simulink model "mcb_open_loop_control_f28035_DRV8312"  (R2021b)
settings: Solver=FixedStepDiscrete  StartTime=0.0  StopTime=Inf  RelTol=1e-3  EnableMultiTasking=on
InitFcn:
  | mcb_c2000_open_loop_control_data;
  | target = mcb_SetProcessorDetails('F28035',PWM_frequency);
model workspace (MAT data in the model file):
  encoderResolution = 2000
  hallOffset = '0.5'
  indexOffset = 850
  polePairs = '4'
values from neighbouring files (symbols this model uses):
  PWM_frequency = 20e3    (= 20000)    [c28027pmsmfoc_data.m]    (also in c28035pmsmfoc_data.m; c28035pmsmfoc_data_cla.m = 12000; c28069pmsmfoc_data.m; mcb_c2000_open_loop_control_data.m = eval(get_param([bdroot '/Open Loop Control/Parameters/PWM Fr)
  Ts = 5e-8    (= 5e-08)    [DCDC_Buck_Param.m]    (also in mcb_c2000_open_loop_control_data.m = T_pwm; mcb_c2000_pmsm_offset_data.m = T_pwm; mcb_pmsm_foc_dual_f28379d_data.m = 5e-05; mcb_pmsm_foc_dual_f28379d_datascript.m = 5e-05)
undefined symbols (not defined in the file or in its folder): DiscIntNeverNeededParam, Down, GPTRIP1SEL, GPTRIP2SEL, motor, TZ1, TZ2, Up
libraries: c2802xlib x4, simulink x3, mcbcontrolslib x3, c2803xlib x2, c280xlib x2, c2000lib x1, demo_controls x1
settings Model: ExtModeTrigDuration=8  Creator=The MathWorks, Inc.  LastModifiedBy=The MathWorks, Inc.
settings SolverCC: AlgebraicLoopSolver=TrustRegion  AutoInsertRateTranBlk=on
settings DataIOCC: LimitDataPoints=on  SaveFormat=Array  SaveOutput=off  SaveTime=off  ReturnWorkspaceOutputs=off
settings OptimizationCC: DefaultParameterBehavior=Inlined  DefaultUnderspecifiedDataType=single  OptimizeBlockIOStorage=off  BufferReuse=off  GlobalBufferReuse=off  ExpressionFolding=off  ExpressionDepthLimit=2147483647  LocalBlockOutputs=off  InitFltsAndDblsToZero=on  NoFixptDivByZeroProtection=on  EfficientFloat2IntCast=on  EfficientMapNaN2IntZero=off  LifeSpan=Inf  MaxStackSize=768  OptimizeDataStoreBuffers=off  BusAssignmentInplaceUpdate=off  DenormalBehavior=FlushToZero  EfficientTunableParamExpr=on
settings DebuggingCC: ReadBeforeWriteMsg=DisableAll  WriteAfterWriteMsg=DisableAll  WriteAfterReadMsg=DisableAll  CheckSSInitialOutputMsg=off  SignalResolutionControl=TryResolveAllWithWarning  SolverPrmCheckMsg=warning  InheritedTsInSrcMsg=none  MultiTaskDSMMsg=none  MultiTaskCondExecSysMsg=none  TasksWithSamePriorityMsg=none  SigSpecEnsureSampleTimeMsg=none  IntegerOverflowMsg=none  ParameterPrecisionLossMsg=none  FcnCallInpInsideContextMsg=warning  AllowSymbolicDim=off  StateNameClashWarn=warning  SFUnexpectedBacktrackingDiag=warning  SFNoUnconditionalDefaultTransitionDiag=warning  SFExecutionAtInitializationDiag=none  SFMachineParentedDataDiag=warning  IntegerSaturationMsg=none  ArithmeticOperatorsInVariantConditions=warning
settings HardwareCC: ProdBitPerChar=16  ProdBitPerInt=16  ProdBitPerPointer=32  ProdBitPerSizeT=32  ProdBitPerPtrDiffT=32  ProdLargestAtomicInteger=Integer  ProdLargestAtomicFloat=None  ProdWordSize=16  ProdLongLongMode=on  ProdHWDeviceType=Texas Instruments->C2000  TargetBitPerChar=16  TargetBitPerInt=16  TargetBitPerPointer=16  TargetLargestAtomicInteger=Integer  TargetIntDivRoundTo=Zero  TargetEndianess=LittleEndian  TargetWordSize=16  TargetHWDeviceType=TI C2000
settings ModelReferenceCC: PropagateSignalLabelsOutOfModel=off
settings SFSimCC: SimUseLocalCustomCode=off  MATLABDynamicMemAlloc=off  CustomCodeUndefinedFunction=UseInterfaceOnly
settings RTWCC: Description=Embedded Coder  SystemTargetFile=ert.tlc  HardwareBoard=TI Piccolo F2803x  TemplateMakefile=ert_default_tmf  GenerateReport=on  RTWUseLocalCustomCode=off  Toolchain=Texas Instruments Code Composer Studio (C2000)  IncludeHyperlinkInReport=on  GenerateTraceInfo=on  GenerateTraceReport=on  GenerateTraceReportSl=on  GenerateTraceReportSf=on  GenerateTraceReportEml=on
settings CodeAppCC: IgnoreCustomStorageClasses=off  CustomSymbolStrType=$N$R$M  StateflowObjectComments=on  InternalIdentifier=Classic
settings ERTTargetCC: CodeReplacementLibrary=TI C28x  MultiwordLength=2048  ExtModeTransport=3  ExtModeStaticAllocSize=1000  ConvertIfToSwitch=off  SuppressUnreachableDefaultCases=off  MemSecPackage=tic2000demospkg
settings ConfigComp: CovMetricSettings=dw  CovSaveCumulativeToWorkspaceVar=on  CovSaveSingleToWorkspaceVar=on  CovExternalEMLEnable=off  CovSFcnEnable=off

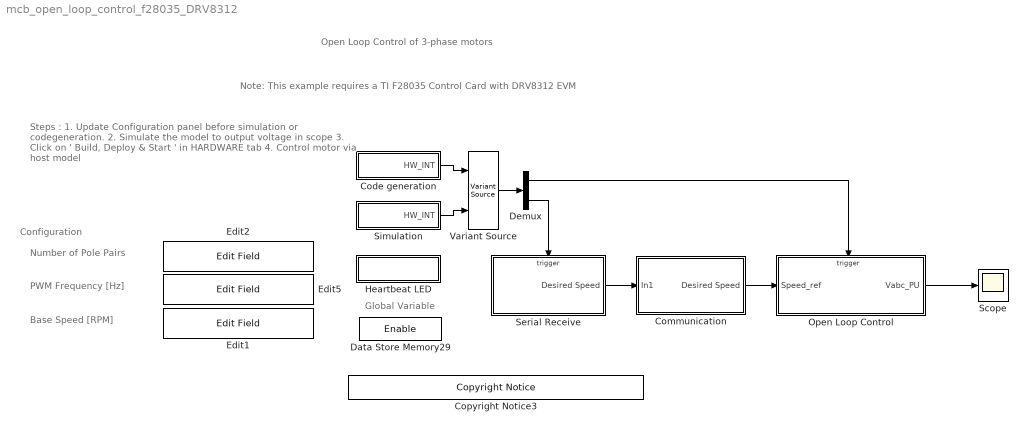
== system mcb_open_loop_control_f28035_DRV8312 ==
  note: Global Variable
  note: Open Loop Control of 3-phase motors
  note: Note: This example requires a TI F28035 Control Card with DRV8312 EVM
  note: Base Speed [RPM]
  note: Number of Pole Pairs
  note: Configuration
  note: PWM Frequency [Hz]
  note: Steps :
      | 1. Update Configuration panel before simulation or
      | codegeneration.
      | 2. Simulate the model to output voltage in scope
      | 3. Click on ' Build, Deploy & Start ' in HARDWARE tab
      | 4. Control motor via host model
  Code generation : Subsystem
  Communication : Subsystem
  Copyright Notice3 : demo_controls/Copyright Notice  year=2021  prod=tic2000
      settings: SourceProductBaseCode=ME
  Data Store Memory29 : DataStoreMemory  DataStoreName=Enable  ShowAdditionalParam=off  OutDataTypeStr=boolean
  Demux : Demux  Outputs=2
  Edit1 : EditField  LabelPosition=Hide  ShowInitialText=on  Alignment=Center
  Edit2 : EditField  LabelPosition=Hide  ShowInitialText=on  Alignment=Center
  Edit5 : EditField  LabelPosition=Hide  ShowInitialText=on  Alignment=Center
  Heartbeat LED : Subsystem  TreatAsAtomicUnit=on
  Open Loop Control : Subsystem
      settings: RTWSystemCode=Nonreusable function
  Scope : Scope
  Serial Receive : Subsystem  SystemSampleTime=1e-3
      settings: RTWSystemCode=Nonreusable function
  Simulation : Subsystem
  Variant Source : VariantSource  VariantControlMode=sim codegen switching  OutputFunctionCall=on
  wires:
  Demux/2 -> Serial Receive/Trigger
  Demux/1 -> Open Loop Control/Trigger
  Open Loop Control/1(Vabc_PU) -> Scope/1
  Code generation/1(HW_INT) -> Variant Source/1
  Simulation/1(HW_INT) -> Variant Source/2
  Variant Source/1 -> Demux/1
  Communication/1(Desired Speed) -> Open Loop Control/1(Speed_ref)
  Serial Receive/1(Desired Speed) -> Communication/1(In1)

== system mcb_open_loop_control_f28035_DRV8312/Code generation ==
  C28x Hardware Interrupt : c2000lib/Scheduling/C28x Hardware Interrupt  irqnumbers=[1 9]  pienumbers=[1 1]  irqpriorities=[30 50]  irqpreempts=[1 0]  showinput=off  dspchiptype=C280X
      settings: SourceProductBaseCode=TIC2000
  HW_INT : Outport
  wires:
  C28x Hardware Interrupt/1 -> HW_INT/1

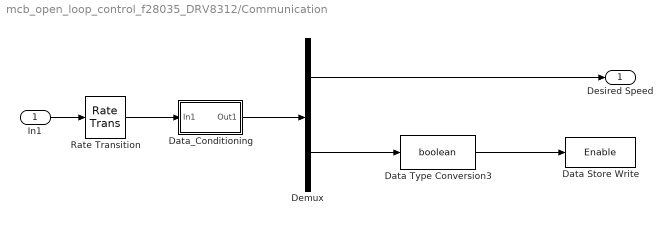
== system mcb_open_loop_control_f28035_DRV8312/Communication ==
  In1 : Inport
  Data Store Write : DataStoreWrite  DataStoreName=Enable  IndexOptions=Index vector (dialog)  Indices=1  OutputSizes=1
  Data Type Conversion3 : DataTypeConversion  OutDataTypeStr=boolean  RndMeth=Simplest
  Data_Conditioning : Subsystem
  Demux : Demux  Outputs=2
  Rate Transition : RateTransition  Deterministic=off  InitialCondition=[1228 0]  OutPortSampleTime=Ts
  Desired Speed : Outport  VectorParamsAs1DForOutWhenUnconnected=off
  wires:
  Rate Transition/1 -> Data_Conditioning/1(In1)
  In1/1 -> Rate Transition/1
  Data_Conditioning/1(Out1) -> Demux/1
  Demux/2 -> Data Type Conversion3/1
  Demux/1 -> Desired Speed/1
  Data Type Conversion3/1 -> Data Store Write/1

== system mcb_open_loop_control_f28035_DRV8312/Heartbeat LED ==
  Code generation : Subsystem
  LED 1 Hz : Constant  OutDataTypeStr=uint16  SampleTime=0.5
  Simulation : Subsystem
  Variant Sink : VariantSink  VariantControlMode=sim codegen switching
  wires:
  Variant Sink/1 -> Code generation/1(In1)
  Variant Sink/2 -> Simulation/1(In1)
  LED 1 Hz/1 -> Variant Sink/1

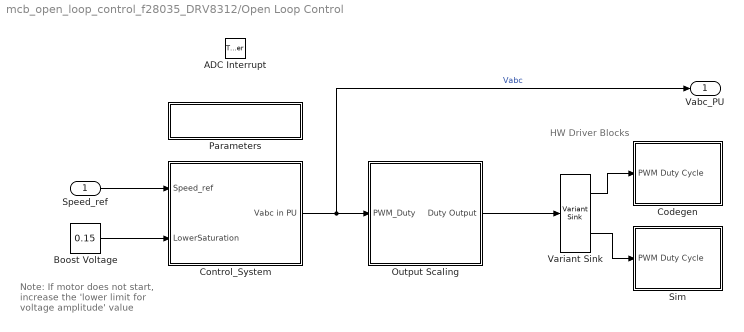
== system mcb_open_loop_control_f28035_DRV8312/Open Loop Control ==
  note: Note: If motor does not start, increase the 'lower limit for voltage amplitude' value
  note: HW Driver Blocks
  Speed_ref : Inport
  ADC Interrupt : TriggerPort  TriggerType=function-call  VariantControl=Variant
  Boost Voltage : Constant  Value=0.15  OutDataTypeStr=dataType
  Codegen : Subsystem
  Control_System : Subsystem
  Output Scaling : Subsystem
  Parameters : Subsystem
  Sim : Subsystem
  Variant Sink : VariantSink  VariantControlMode=sim codegen switching
  Vabc_PU : Outport  VectorParamsAs1DForOutWhenUnconnected=off
  wires:
  Speed_ref/1 -> Control_System/1(Speed_ref)
  Control_System/1(Vabc in PU) -> Vabc_PU/1, Output Scaling/1(PWM_Duty)  "Vabc"
  Output Scaling/1(Duty Output) -> Variant Sink/1
  Variant Sink/1 -> Codegen/1(PWM Duty Cycle)
  Variant Sink/2 -> Sim/1(PWM Duty Cycle)
  Boost Voltage/1 -> Control_System/2(LowerSaturation)

== system mcb_open_loop_control_f28035_DRV8312/Serial Receive ==
  SCI_Rx_INT : TriggerPort  TriggerType=function-call  VariantControl=Variant
  Codegen : Subsystem
  Sim : Subsystem
  Variant Source : VariantSource  VariantControlMode=sim codegen switching
  Desired Speed : Outport  VectorParamsAs1DForOutWhenUnconnected=off
  wires:
  Variant Source/1 -> Desired Speed/1
  Codegen/1(Output) -> Variant Source/1
  Sim/1(Out1) -> Variant Source/2

== system mcb_open_loop_control_f28035_DRV8312/Simulation ==
  ADCINT1 : simulink/Ports & Subsystems/Function-Call Generator  sample_time=Ts  numberOfIterations=1  DisallowWideOutput=off
  Mux : Mux  Inputs=2
  SCI_Rx_INT : simulink/Ports & Subsystems/Function-Call Generator  sample_time=0.1  numberOfIterations=1  DisallowWideOutput=off
  HW_INT : Outport
  wires:
  SCI_Rx_INT/1 -> Mux/2
  ADCINT1/1 -> Mux/1
  Mux/1 -> HW_INT/1

== system mcb_open_loop_control_f28035_DRV8312/Communication/Data_Conditioning ==
  In1 : Inport
  Data Type Conversion2 : DataTypeConversion  OutDataTypeStr=int16  ConvertRealWorld=Stored Integer (SI)  RndMeth=Simplest
  Out1 : Outport  VectorParamsAs1DForOutWhenUnconnected=off
  wires:
  Data Type Conversion2/1 -> Out1/1
  In1/1 -> Data Type Conversion2/1

== system mcb_open_loop_control_f28035_DRV8312/Heartbeat LED/Code generation ==
  In1 : Inport
  Digital Output1 : c2803xlib/Digital Output  GPIO_Number=GPIO24~GPIO31  GPIO_Bit0=off  GPIO_BIT0_Toggle=off  GPIO_Bit1=off  GPIO_BIT1_Toggle=off  GPIO_Bit2=off  GPIO_BIT2_Toggle=off  GPIO_Bit3=off  GPIO_BIT3_Toggle=off  GPIO_Bit4=off  GPIO_BIT4_Toggle=off  GPIO_Bit5=off  GPIO_BIT5_Toggle=off  GPIO_Bit6=off  GPIO_BIT6_Toggle=off  GPIO_Bit7=on  GPIO_BIT7_Toggle=on
      settings: SourceProductBaseCode=TIC2000
  wires:
  In1/1 -> Digital Output1/1

== system mcb_open_loop_control_f28035_DRV8312/Heartbeat LED/Simulation ==
  In1 : Inport
  Simulation_Terminator : Terminator
  wires:
  In1/1 -> Simulation_Terminator/1

== system mcb_open_loop_control_f28035_DRV8312/Open Loop Control/Codegen ==
  PWM Duty Cycle : Inport
  Data Serial Output : Subsystem
  Demux : Demux  Outputs=2
  Hardware Initialization : Subsystem
  PWM Output : Subsystem
  Sensors : Subsystem
  wires:
  Demux/2 -> Data Serial Output/2(Data2_Log)
  Sensors/1(Iab_measured_ADC) -> Demux/1
  Demux/1 -> Data Serial Output/1(Data1_Log)
  PWM Duty Cycle/1 -> PWM Output/1(PWM Duty Cycle)

== system mcb_open_loop_control_f28035_DRV8312/Open Loop Control/Control_System ==
  Speed_ref : Inport
  LowerSaturation : Inport  Port=2
  SpeedRefToFreq : Subsystem
  VabcCalc : Subsystem
  Vabc in PU : Outport  VectorParamsAs1DForOutWhenUnconnected=off
  wires:
  Speed_ref/1 -> SpeedRefToFreq/1(Speed_Ref)
  SpeedRefToFreq/1(Frequency) -> VabcCalc/1(Frequency)
  VabcCalc/1(Vabc) -> Vabc in PU/1
  LowerSaturation/1 -> VabcCalc/2(LowerSaturation)

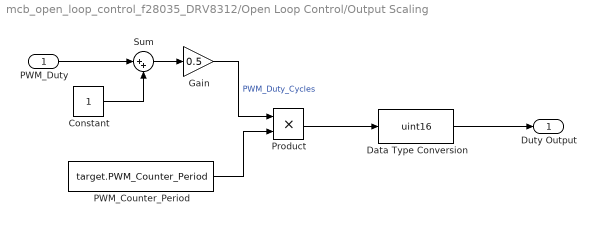
== system mcb_open_loop_control_f28035_DRV8312/Open Loop Control/Output Scaling ==
  PWM_Duty : Inport
  Constant : Constant  OutDataTypeStr=dataType
  Data Type Conversion : DataTypeConversion  OutDataTypeStr=uint16  SaturateOnIntegerOverflow=on
  Gain : Gain  Gain=0.5  RndMeth=Simplest  OutDataTypeStr=Inherit: Same as input
  PWM_Counter_Period : Constant  Value=target.PWM_Counter_Period  OutDataTypeStr=dataType  SampleTime=-1
  Product : Product  RndMeth=Simplest  OutDataTypeStr=Inherit: Same as first input
  Sum : Sum  Inputs=|++
  Duty Output : Outport
  wires:
  Data Type Conversion/1 -> Duty Output/1
  PWM_Counter_Period/1 -> Product/2
  PWM_Duty/1 -> Sum/1
  Product/1 -> Data Type Conversion/1
  Constant/1 -> Sum/2
  Sum/1 -> Gain/1
  Gain/1 -> Product/1  "PWM_Duty_Cycles"

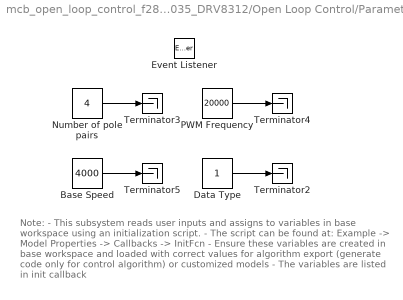
== system mcb_open_loop_control_f28035_DRV8312/Open Loop Control/Parameters ==
  note: Note:
      | - This subsystem reads user inputs and assigns to variables
      | in base workspace using an initialization script.
      | - The script can be found at: Example -> Model Properties ->
      | Callbacks -> InitFcn
      | - Ensure these variables are created in base workspace and
      | loaded with correct values for algorithm export (generate
      | code only for control algorithm) or customized models
      | - The variables are listed in init callback
  Base Speed : Constant  Value=4000
  Data Type : Constant
  Event Listener : EventListener  DisableCoverage=on  EventName=reset
  Number of pole pairs : Constant  Value=4
  PWM Frequency : Constant  Value=20000
  Terminator{2..5} (4 alike) : Terminator
  wires:
  Data Type/1 -> Terminator2/1
  Number of pole pairs/1 -> Terminator3/1
  PWM Frequency/1 -> Terminator4/1
  Base Speed/1 -> Terminator5/1

== system mcb_open_loop_control_f28035_DRV8312/Open Loop Control/Sim ==
  PWM Duty Cycle : Inport
  Terminator : Terminator
  wires:
  PWM Duty Cycle/1 -> Terminator/1

== system mcb_open_loop_control_f28035_DRV8312/Serial Receive/Codegen ==
  SCI Receive : c280xlib/SCI Receive  sciModule=A  dataHead=''  dataTail=''  dataType=uint16  dataDim=2  initValue=0  errOption=Output the last received value  errValue=0  sampleTime=-1  outputStatus=off  postInterrupt=on  numFifo=4
      settings: SourceProductBaseCode=TIC2000
  Output : Outport
  wires:
  SCI Receive/1 -> Output/1

== system mcb_open_loop_control_f28035_DRV8312/Serial Receive/Sim ==
  Constant : Constant  OutDataTypeStr=dataType
  Data Type Conversion : DataTypeConversion  OutDataTypeStr=int16
  Data Type Conversion3 : DataTypeConversion  OutDataTypeStr=uint16  ConvertRealWorld=Stored Integer (SI)  RndMeth=Simplest
  Mux : Mux  Inputs=2
  Speed_ref_rpm (sim) : Constant  Value=1200  OutDataTypeStr=dataType  SampleTime=-1
  Out1 : Outport
  wires:
  Data Type Conversion3/1 -> Out1/1
  Mux/1 -> Data Type Conversion/1
  Constant/1 -> Mux/2
  Speed_ref_rpm (sim)/1 -> Mux/1
  Data Type Conversion/1 -> Data Type Conversion3/1

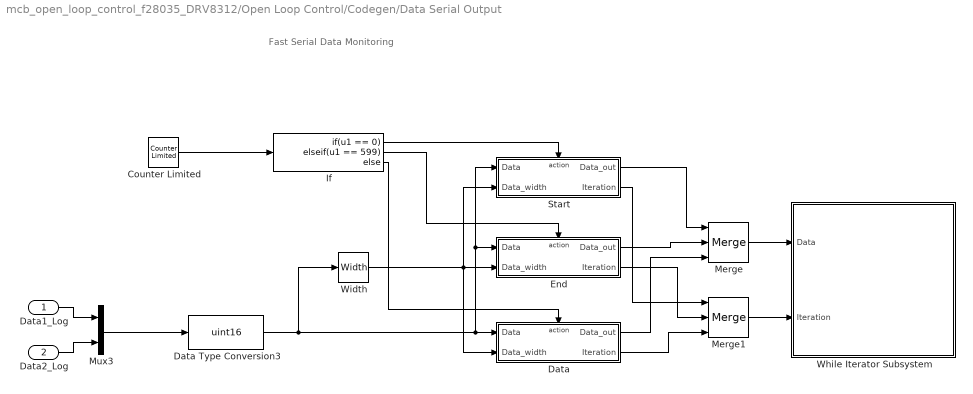
== system mcb_open_loop_control_f28035_DRV8312/Open Loop Control/Codegen/Data Serial Output ==
  note: Fast Serial Data Monitoring
  Data1_Log : Inport
  Data2_Log : Inport  Port=2
  Counter Limited : simulink/Sources/Counter Limited  uplimit=599  tsamp=-1
  Data : Subsystem  TreatAsAtomicUnit=on
  Data Type Conversion3 : DataTypeConversion  OutDataTypeStr=uint16  ConvertRealWorld=Stored Integer (SI)
  End : Subsystem  TreatAsAtomicUnit=on
  If : If  IfExpression=u1 == 0  ElseIfExpressions=u1 == 599
  Merge : Merge  Inputs=3
  Merge1 : Merge  Inputs=3
  Mux3 : Mux  Inputs=2
  Start : Subsystem  TreatAsAtomicUnit=on
  While Iterator Subsystem : Subsystem  TreatAsAtomicUnit=on
  Width : Width  OutDataTypeMode=All ports same datatype  DataType=uint16
  wires:
  Merge/1 -> While Iterator Subsystem/1(Data)
  If/2 -> End/Action
  If/3 -> Data/Action
  Counter Limited/1 -> If/1
  End/1(Data_out) -> Merge/2
  Width/1 -> Data/2(Data_width), Start/2(Data_width), End/2(Data_width)
  Start/1(Data_out) -> Merge/1
  Start/2(Iteration) -> Merge1/1
  Merge1/1 -> While Iterator Subsystem/2(Iteration)
  Data/1(Data_out) -> Merge/3
  If/1 -> Start/Action
  End/2(Iteration) -> Merge1/2
  Data/2(Iteration) -> Merge1/3
  Data Type Conversion3/1 -> Width/1, Start/1(Data), End/1(Data), Data/1(Data)
  Data2_Log/1 -> Mux3/2
  Data1_Log/1 -> Mux3/1
  Mux3/1 -> Data Type Conversion3/1

== system mcb_open_loop_control_f28035_DRV8312/Open Loop Control/Codegen/Hardware Initialization ==
  Data Store Read1 : DataStoreRead  DataStoreName=Enable  IndexOptions=Index vector (dialog)  Indices=1  OutputSizes=1
  Digital Output : c2803xlib/Digital Output  GPIO_Number=GPIO0~GPIO7  GPIO_Bit0=off  GPIO_BIT0_Toggle=off  GPIO_Bit1=on  GPIO_BIT1_Toggle=off  GPIO_Bit2=off  GPIO_BIT2_Toggle=off  GPIO_Bit3=on  GPIO_BIT3_Toggle=off  GPIO_Bit4=off  GPIO_BIT4_Toggle=off  GPIO_Bit5=on  GPIO_BIT5_Toggle=off  GPIO_Bit6=off  GPIO_BIT6_Toggle=off  GPIO_Bit7=off  GPIO_BIT7_Toggle=off
      settings: SourceProductBaseCode=TIC2000
  Mux : Mux  Inputs=3
  wires:
  Mux/1 -> Digital Output/1
  Data Store Read1/1 -> Mux/3, Mux/2, Mux/1

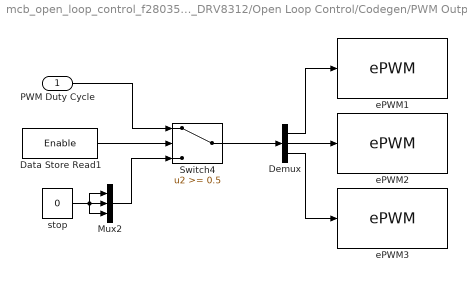
== system mcb_open_loop_control_f28035_DRV8312/Open Loop Control/Codegen/PWM Output ==
  PWM Duty Cycle : Inport
  Data Store Read1 : DataStoreRead  DataStoreName=Enable  IndexOptions=Index vector (dialog)  Indices=1  OutputSizes=1
  Demux : Demux  Outputs=3
  Mux2 : Mux  Inputs=3
  Switch4 : Switch  Threshold=0.5  RndMeth=Simplest
  ePWM1 : c2802xlib/ePWM  PwmType=C2000  useModule=ePWM1  ePWMxLINKTBPRD=Not Linked  periodUnits=Clock cycles  timerSource=Specify via dialog  timerPeriod_clk=target.PWM_Counter_Period+1  timerPeriod_sec=64000  tbshadow=Counter equals to zero  countingMode=Up-Down  phaseActiveEnable=Disable  phaseDirection=Count down after sync  phaseActive=0  synchronizationEnable=off  dcaevt1Sync=off  dcbevt1Sync=off  synchronizationOption=Counter equals to zero (CTR=Zero)  perSynchronizationOption=Counter equals to period (CTR=PRD)  clockPrescale=1  HSclockPrescale=1  enswap=off  ePWMxAStatus=on  ePWMxAactionLogic1=Do nothing  ePWMxAactionLogic2=Do nothing  ePWMxAactionLogic3=Clear  ePWMxAactionLogic4=Set  ePWMxAactionLogic5=Do nothing  ePWMxAactionLogic6=Do nothing  ePWMxACSFenable=off  ePWMxACSFvalue=Forcing disable  ePWMxASFreload=Zero  ePWMxBStatus=off  ePWMxBactionLogic1=Do nothing  ePWMxBactionLogic2=Set  ePWMxBactionLogic3=Do nothing  ePWMxBactionLogic4=Do nothing  ePWMxBactionLogic5=Clear  ePWMxBactionLogic6=Do nothing  ePWMxBCSFenable=off  ePWMxBCSFvalue=Forcing disable  ePWMxBSFreload=Zero  ePWNxBOutWay=off  ePWMxLINKCMPA=Not Linked  CMPAUnits=Clock cycles  CMPASource=Input port  CMPAValue_per=32000  CMPAValue_clk=target.PWM_Counter_Period/2+1  enCMPAshadow=Counter equals to zero (CTR=Zero)  ePWMxLINKCMPB=Not Linked  CMPBUnits=Clock cycles  CMPBSource=Specify via dialog  CMPBValue_per=50  CMPBValue_clk=target.PWM_Counter_Period/2+1  enCMPBshadow=Counter equals to zero (CTR=Zero)  ePWMxLINKCMPC=Not Linked  CMPCUnits=Clock cycles  CMPCSource=Specify via dialog  CMPCValue_per=50  CMPCValue_clk=32000  enCMPCshadow=Counter equals to zero (CTR=Zero)  ePWMxLINKCMPD=Not Linked  CMPDUnits=Clock cycles  CMPDSource=Specify via dialog  CMPDValue_per=50  CMPDValue_clk=32000  enCMPDshadow=Counter equals to zero (CTR=Zero)  enableDBePWMxA=off  enableDBePWMxB=off  enhalfcycle=off  DBpolarity=Active high (AH)  DBedgeDelay=Positive  DBSource_ePWMxA=ePWMxA  DBSource_ePWMxB=ePWMxA  DBPeriodUnits=Clock cycles  DBperiodSource=Specify via dialog  REDperiod=0  FEDperiod=0  REDperiod_sec=0  FEDperiod_sec=0  LoadModeDBRED=Immediate without using shadow  LoadModeDBFED=Immediate without using shadow  adcstartModuleA=on  adcrequestEventA=First event  adcstartEventA=Counter equals to period (CTR=PRD)  adcstartEventA_type2=Digital Compare Module A Event 1 start of conversion (DCAEVT1.soc)  adcstartModuleB=off  adcrequestEventB=First event  adcstartEventB=Counter equals to zero (CTR=Zero)  adcstartEventB_type2=Counter equals to zero (CTR=Zero)  intEn=off  intPrd=First event  intSel=Counter equals to zero (CTR=Zero)  intSel_type2=Counter equals to zero (CTR=Zero)  hrpe=off  enHRPWM=off  HRPWM_LoadMode=Counter equals to period (CTR=PRD)  HRPWM_CTLMode=Duty or Period control mode  HRPWM_EDGMode=Both edge  hrpeb=off  enHRPWMB=off  HRPWM_LoadModeB=Counter equals to zero (CTR=ZERO)  HRPWM_CTLModeB=Duty or Period control mode  HRPWM_EDGModeB=Both edge  enHRDBRED=off  enHRDBFED=off  enSFO=on  enautoconv=on  chopperEnable=off  chopperFrequency=1  chopperFirstwidth=1  chopperDuty=12.5%  tripZonesource=Specify via dialog  tzselOSHT1=off  tzselOSHT2=off  tzselOSHT3=off  tzselOSHDCAEV1=off  tzselOSHDCBEV1=off  tzselCBC1=off  tzselCBC2=off  tzselCBC3=off  tzselCBCDCAEV2=off  tzselCBCDCBEV2=off  tzselOSHT4=off  tzselOSHT5=off  tzselOSHT6=off  tzselCBC4=off  tzselCBC5=off  tzselCBC6=off  enTzOstIntr=off  enTzCbcIntr=off  enTzDCAEVT1Intr=off  enTzDCAEVT2Intr=off  enTzDCBEVT1Intr=off  enTzDCBEVT2Intr=off  ePWMxAforced=No action  ePWMxBforced=No action  DCAEVT1forced=No action  DCBEVT1forced=No action  DCAEVT2forced=No action  DCBEVT2forced=No action  dcah=Trip Zone 1 input (TZ1)  dcal=Trip Zone 2 input (TZ2)  dcbh=Trip Zone 1 input (TZ1)  dcbl=Trip Zone 2 input (TZ2)  dcah_type2=GPTRIP1SEL/(TZ1)  dcal_type2=GPTRIP2SEL/(TZ2)  dcbh_type2=GPTRIP1SEL/(TZ1)  dcbl_type2=GPTRIP2SEL/(TZ2)  gendcaevt1=Event disabled  gendcaevt2=Event disabled  gendcbevt1=Event disabled  gendcbevt2=Event disabled  dcaevt1src=DCAEVT1 with sync  dcaevt2src=DCAEVT2 with sync  dcbevt1src=DCBEVT1 with sync  dcbevt2src=DCBEVT2 with sync  pulsesel=Counter equals to zero (CTR=Zero)  blankinv=off  blankoffset=0  blankwidth=0  evsrcsel=Filtered version of DCAEVT1 (DCAEVT1FILT)  encape=off
  ePWM2 : c2802xlib/ePWM  PwmType=C2000  useModule=ePWM2  ePWMxLINKTBPRD=Not Linked  periodUnits=Clock cycles  timerSource=Specify via dialog  timerPeriod_clk=target.PWM_Counter_Period+1  timerPeriod_sec=64000  tbshadow=Counter equals to zero  countingMode=Up-Down  phaseActiveEnable=Set counter to phase value specified via dialog  phaseDirection=Count up after sync  phaseActive=0  synchronizationEnable=off  dcaevt1Sync=off  dcbevt1Sync=off  synchronizationOption=Pass through (EPWMxSYNCI or SWFSYNC)  perSynchronizationOption=Counter equals to period (CTR=PRD)  clockPrescale=1  HSclockPrescale=1  enswap=off  ePWMxAStatus=on  ePWMxAactionLogic1=Do nothing  ePWMxAactionLogic2=Do nothing  ePWMxAactionLogic3=Clear  ePWMxAactionLogic4=Set  ePWMxAactionLogic5=Do nothing  ePWMxAactionLogic6=Do nothing  ePWMxACSFenable=off  ePWMxACSFvalue=Forcing disable  ePWMxASFreload=Zero  ePWMxBStatus=off  ePWMxBactionLogic1=Do nothing  ePWMxBactionLogic2=Set  ePWMxBactionLogic3=Do nothing  ePWMxBactionLogic4=Do nothing  ePWMxBactionLogic5=Clear  ePWMxBactionLogic6=Do nothing  ePWMxBCSFenable=off  ePWMxBCSFvalue=Forcing disable  ePWMxBSFreload=Zero  ePWNxBOutWay=off  ePWMxLINKCMPA=Not Linked  CMPAUnits=Clock cycles  CMPASource=Input port  CMPAValue_per=32000  CMPAValue_clk=target.PWM_Counter_Period/2+1  enCMPAshadow=Counter equals to zero (CTR=Zero)  ePWMxLINKCMPB=Not Linked  CMPBUnits=Clock cycles  CMPBSource=Specify via dialog  CMPBValue_per=50  CMPBValue_clk=target.PWM_Counter_Period/2+1  enCMPBshadow=Counter equals to zero (CTR=Zero)  ePWMxLINKCMPC=Not Linked  CMPCUnits=Clock cycles  CMPCSource=Specify via dialog  CMPCValue_per=50  CMPCValue_clk=32000  enCMPCshadow=Counter equals to zero (CTR=Zero)  ePWMxLINKCMPD=Not Linked  CMPDUnits=Clock cycles  CMPDSource=Specify via dialog  CMPDValue_per=50  CMPDValue_clk=32000  enCMPDshadow=Counter equals to zero (CTR=Zero)  enableDBePWMxA=off  enableDBePWMxB=off  enhalfcycle=off  DBpolarity=Active high (AH)  DBedgeDelay=Positive  DBSource_ePWMxA=ePWMxA  DBSource_ePWMxB=ePWMxA  DBPeriodUnits=Clock cycles  DBperiodSource=Specify via dialog  REDperiod=0  FEDperiod=0  REDperiod_sec=0  FEDperiod_sec=0  LoadModeDBRED=Immediate without using shadow  LoadModeDBFED=Immediate without using shadow  adcstartModuleA=off  adcrequestEventA=First event  adcstartEventA=Digital Compare Module A Event 1 start of conversion (DCAEVT1.soc)  adcstartEventA_type2=Digital Compare Module A Event 1 start of conversion (DCAEVT1.soc)  adcstartModuleB=off  adcrequestEventB=First event  adcstartEventB=Counter equals to zero (CTR=Zero)  adcstartEventB_type2=Counter equals to zero (CTR=Zero)  intEn=off  intPrd=First event  intSel=Counter equals to zero (CTR=Zero)  intSel_type2=Counter equals to zero (CTR=Zero)  hrpe=off  enHRPWM=off  HRPWM_LoadMode=Counter equals to period (CTR=PRD)  HRPWM_CTLMode=Duty or Period control mode  HRPWM_EDGMode=Both edge  hrpeb=off  enHRPWMB=off  HRPWM_LoadModeB=Counter equals to zero (CTR=ZERO)  HRPWM_CTLModeB=Duty or Period control mode  HRPWM_EDGModeB=Both edge  enHRDBRED=off  enHRDBFED=off  enSFO=on  enautoconv=on  chopperEnable=off  chopperFrequency=1  chopperFirstwidth=1  chopperDuty=12.5%  tripZonesource=Specify via dialog  tzselOSHT1=off  tzselOSHT2=off  tzselOSHT3=off  tzselOSHDCAEV1=off  tzselOSHDCBEV1=off  tzselCBC1=off  tzselCBC2=off  tzselCBC3=off  tzselCBCDCAEV2=off  tzselCBCDCBEV2=off  tzselOSHT4=off  tzselOSHT5=off  tzselOSHT6=off  tzselCBC4=off  tzselCBC5=off  tzselCBC6=off  enTzOstIntr=off  enTzCbcIntr=off  enTzDCAEVT1Intr=off  enTzDCAEVT2Intr=off  enTzDCBEVT1Intr=off  enTzDCBEVT2Intr=off  ePWMxAforced=No action  ePWMxBforced=No action  DCAEVT1forced=No action  DCBEVT1forced=No action  DCAEVT2forced=No action  DCBEVT2forced=No action  dcah=Trip Zone 1 input (TZ1)  dcal=Trip Zone 2 input (TZ2)  dcbh=Trip Zone 1 input (TZ1)  dcbl=Trip Zone 2 input (TZ2)  dcah_type2=GPTRIP1SEL/(TZ1)  dcal_type2=GPTRIP2SEL/(TZ2)  dcbh_type2=GPTRIP1SEL/(TZ1)  dcbl_type2=GPTRIP2SEL/(TZ2)  gendcaevt1=Event disabled  gendcaevt2=Event disabled  gendcbevt1=Event disabled  gendcbevt2=Event disabled  dcaevt1src=DCAEVT1 with sync  dcaevt2src=DCAEVT2 with sync  dcbevt1src=DCBEVT1 with sync  dcbevt2src=DCBEVT2 with sync  pulsesel=Counter equals to zero (CTR=Zero)  blankinv=off  blankoffset=0  blankwidth=0  evsrcsel=Filtered version of DCAEVT1 (DCAEVT1FILT)  encape=off
  ePWM3 : c2802xlib/ePWM  PwmType=C2000  useModule=ePWM3  ePWMxLINKTBPRD=Not Linked  periodUnits=Clock cycles  timerSource=Specify via dialog  timerPeriod_clk=target.PWM_Counter_Period+1  timerPeriod_sec=64000  tbshadow=Counter equals to zero  countingMode=Up-Down  phaseActiveEnable=Set counter to phase value specified via dialog  phaseDirection=Count up after sync  phaseActive=0  synchronizationEnable=off  dcaevt1Sync=off  dcbevt1Sync=off  synchronizationOption=Disable  perSynchronizationOption=Counter equals to period (CTR=PRD)  clockPrescale=1  HSclockPrescale=1  enswap=off  ePWMxAStatus=on  ePWMxAactionLogic1=Do nothing  ePWMxAactionLogic2=Do nothing  ePWMxAactionLogic3=Clear  ePWMxAactionLogic4=Set  ePWMxAactionLogic5=Do nothing  ePWMxAactionLogic6=Do nothing  ePWMxACSFenable=off  ePWMxACSFvalue=Forcing disable  ePWMxASFreload=Zero  ePWMxBStatus=off  ePWMxBactionLogic1=Do nothing  ePWMxBactionLogic2=Set  ePWMxBactionLogic3=Do nothing  ePWMxBactionLogic4=Do nothing  ePWMxBactionLogic5=Clear  ePWMxBactionLogic6=Do nothing  ePWMxBCSFenable=off  ePWMxBCSFvalue=Forcing disable  ePWMxBSFreload=Zero  ePWNxBOutWay=off  ePWMxLINKCMPA=Not Linked  CMPAUnits=Clock cycles  CMPASource=Input port  CMPAValue_per=32000  CMPAValue_clk=target.PWM_Counter_Period/2+1  enCMPAshadow=Counter equals to zero (CTR=Zero)  ePWMxLINKCMPB=Not Linked  CMPBUnits=Clock cycles  CMPBSource=Specify via dialog  CMPBValue_per=50  CMPBValue_clk=target.PWM_Counter_Period/2+1  enCMPBshadow=Counter equals to zero (CTR=Zero)  ePWMxLINKCMPC=Not Linked  CMPCUnits=Clock cycles  CMPCSource=Specify via dialog  CMPCValue_per=50  CMPCValue_clk=32000  enCMPCshadow=Counter equals to zero (CTR=Zero)  ePWMxLINKCMPD=Not Linked  CMPDUnits=Clock cycles  CMPDSource=Specify via dialog  CMPDValue_per=50  CMPDValue_clk=32000  enCMPDshadow=Counter equals to zero (CTR=Zero)  enableDBePWMxA=off  enableDBePWMxB=off  enhalfcycle=off  DBpolarity=Active high (AH)  DBedgeDelay=Positive  DBSource_ePWMxA=ePWMxA  DBSource_ePWMxB=ePWMxA  DBPeriodUnits=Clock cycles  DBperiodSource=Specify via dialog  REDperiod=0  FEDperiod=0  REDperiod_sec=0  FEDperiod_sec=0  LoadModeDBRED=Immediate without using shadow  LoadModeDBFED=Immediate without using shadow  adcstartModuleA=off  adcrequestEventA=First event  adcstartEventA=Digital Compare Module A Event 1 start of conversion (DCAEVT1.soc)  adcstartEventA_type2=Digital Compare Module A Event 1 start of conversion (DCAEVT1.soc)  adcstartModuleB=off  adcrequestEventB=First event  adcstartEventB=Counter equals to zero (CTR=Zero)  adcstartEventB_type2=Counter equals to zero (CTR=Zero)  intEn=off  intPrd=First event  intSel=Counter equals to zero (CTR=Zero)  intSel_type2=Counter equals to zero (CTR=Zero)  hrpe=off  enHRPWM=off  HRPWM_LoadMode=Counter equals to period (CTR=PRD)  HRPWM_CTLMode=Duty or Period control mode  HRPWM_EDGMode=Both edge  hrpeb=off  enHRPWMB=off  HRPWM_LoadModeB=Counter equals to zero (CTR=ZERO)  HRPWM_CTLModeB=Duty or Period control mode  HRPWM_EDGModeB=Both edge  enHRDBRED=off  enHRDBFED=off  enSFO=on  enautoconv=on  chopperEnable=off  chopperFrequency=1  chopperFirstwidth=1  chopperDuty=12.5%  tripZonesource=Specify via dialog  tzselOSHT1=off  tzselOSHT2=off  tzselOSHT3=off  tzselOSHDCAEV1=off  tzselOSHDCBEV1=off  tzselCBC1=off  tzselCBC2=off  tzselCBC3=off  tzselCBCDCAEV2=off  tzselCBCDCBEV2=off  tzselOSHT4=off  tzselOSHT5=off  tzselOSHT6=off  tzselCBC4=off  tzselCBC5=off  tzselCBC6=off  enTzOstIntr=off  enTzCbcIntr=off  enTzDCAEVT1Intr=off  enTzDCAEVT2Intr=off  enTzDCBEVT1Intr=off  enTzDCBEVT2Intr=off  ePWMxAforced=No action  ePWMxBforced=No action  DCAEVT1forced=No action  DCBEVT1forced=No action  DCAEVT2forced=No action  DCBEVT2forced=No action  dcah=Trip Zone 1 input (TZ1)  dcal=Trip Zone 2 input (TZ2)  dcbh=Trip Zone 1 input (TZ1)  dcbl=Trip Zone 2 input (TZ2)  dcah_type2=GPTRIP1SEL/(TZ1)  dcal_type2=GPTRIP2SEL/(TZ2)  dcbh_type2=GPTRIP1SEL/(TZ1)  dcbl_type2=GPTRIP2SEL/(TZ2)  gendcaevt1=Event disabled  gendcaevt2=Event disabled  gendcbevt1=Event disabled  gendcbevt2=Event disabled  dcaevt1src=DCAEVT1 with sync  dcaevt2src=DCAEVT2 with sync  dcbevt1src=DCBEVT1 with sync  dcbevt2src=DCBEVT2 with sync  pulsesel=Counter equals to zero (CTR=Zero)  blankinv=off  blankoffset=0  blankwidth=0  evsrcsel=Filtered version of DCAEVT1 (DCAEVT1FILT)  encape=off
  stop : Constant  Value=0  OutDataTypeStr=single
  wires:
  Demux/3 -> ePWM3/1
  Demux/2 -> ePWM2/1
  PWM Duty Cycle/1 -> Switch4/1
  Demux/1 -> ePWM1/1
  stop/1 -> Mux2/3, Mux2/2, Mux2/1
  Switch4/1 -> Demux/1
  Mux2/1 -> Switch4/3
  Data Store Read1/1 -> Switch4/2

== system mcb_open_loop_control_f28035_DRV8312/Open Loop Control/Codegen/Sensors ==
  Data Type Conversion : DataTypeConversion  OutDataTypeStr=int32  ConvertRealWorld=Stored Integer (SI)
  IA/IB Measurement : c2802xlib/ADC  blkParamProc=C2000  ADCModule=1  samplingMode=Simultaneous sample mode  ADCResolution=12-bit (Single-ended input)  useSOC1=SOC0  useSOC2=SOC0_SOC1  SOCAcquisitionWindow=7  SOCTriggerSource=ePWM1_ADCSOCA  SOCInterruptTrigger=No ADCINT  Ts=-1  dType=uint16  postInterrupt=on  interruptSel=ADCINT1  ADCINTContinuous=on  endma=off  chdma=1  conv1=ADCINA0  conv2=ADCINA1 and ADCINB1  conv1_Type4=ADCIN0  conv2_Type4=ADCIN0 and ADCIN1
  Iab_measured_ADC : Outport  InitialOutput=0  VectorParamsAs1DForOutWhenUnconnected=off
  wires:
  Data Type Conversion/1 -> Iab_measured_ADC/1
  IA/IB Measurement/1 -> Data Type Conversion/1

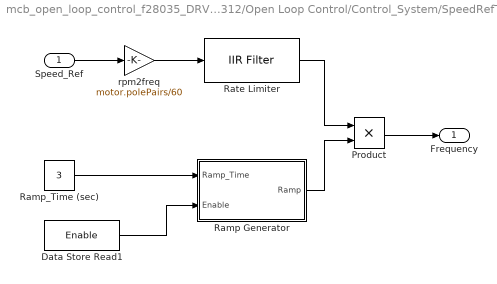
== system mcb_open_loop_control_f28035_DRV8312/Open Loop Control/Control_System/SpeedRefToFreq ==
  Speed_Ref : Inport
  Data Store Read1 : DataStoreRead  DataStoreName=Enable  IndexOptions=Index vector (dialog)  Indices=1  OutputSizes=1
  Product : Product  RndMeth=Simplest  OutDataTypeStr=Inherit: Same as first input
  Ramp Generator : Subsystem
  Ramp_Time (sec) : Constant  Value=3  OutDataTypeStr=dataType  SampleTime=-1
  Rate Limiter : mcbcontrolslib/IIR Filter  VariantControl=Low Pass Filter  VariantSelect=Low-pass  Filter_constant=0.0001  advancedSettings=off  Ts=50e-6  cutOff_freq=0.31834
      settings: SourceProductBaseCode=MT
  rpm2freq : Gain  Gain=motor.polePairs/60  OutDataTypeStr=dataType  RndMeth=Simplest
  Frequency : Outport
  wires:
  Speed_Ref/1 -> rpm2freq/1
  Data Store Read1/1 -> Ramp Generator/2(Enable)
  Product/1 -> Frequency/1
  Ramp Generator/1(Ramp) -> Product/2
  Ramp_Time (sec)/1 -> Ramp Generator/1(Ramp_Time)
  rpm2freq/1 -> Rate Limiter/1
  Rate Limiter/1 -> Product/1

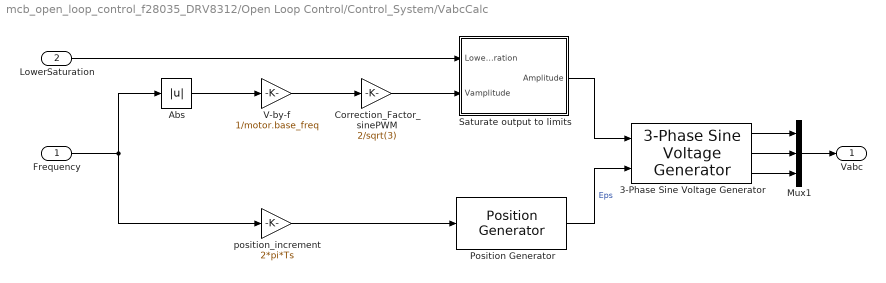
== system mcb_open_loop_control_f28035_DRV8312/Open Loop Control/Control_System/VabcCalc ==
  Frequency : Inport
  LowerSaturation : Inport  Port=2
  3-Phase Sine Voltage Generator : mcbcontrolslib/3-Phase Sine Voltage Generator  AngleInput=Radians  N_points=1024
      settings: SourceProductBaseCode=MT
  Abs : Abs  RndMeth=Simplest
  Correction_Factor_sinePWM : Gain  Gain=2/sqrt(3)  RndMeth=Simplest  OutDataTypeStr=Inherit: Same as input
  Mux1 : Mux  Inputs=3
  Position Generator : mcbcontrolslib/Position Generator  AngleOutput=Radians  ThetaSource=External  ThetaInput=5e-4  DataType=double  ExternalReset=none  Offset=0
      settings: SourceProductBaseCode=MT
  Saturate output to limits : Subsystem
  V-by-f : Gain  Gain=1/motor.base_freq  RndMeth=Simplest  OutDataTypeStr=Inherit: Same as input
  position_increment : Gain  Gain=2*pi*Ts  RndMeth=Simplest  OutDataTypeStr=Inherit: Same as input
  Vabc : Outport
  wires:
  Frequency/1 -> Abs/1, position_increment/1
  3-Phase Sine Voltage Generator/1 -> Mux1/1
  3-Phase Sine Voltage Generator/2 -> Mux1/2
  3-Phase Sine Voltage Generator/3 -> Mux1/3
  position_increment/1 -> Position Generator/1
  Mux1/1 -> Vabc/1
  V-by-f/1 -> Correction_Factor_sinePWM/1
  LowerSaturation/1 -> Saturate output to limits/1(Lower Saturation)
  Saturate output to limits/1(Amplitude) -> 3-Phase Sine Voltage Generator/1
  Correction_Factor_sinePWM/1 -> Saturate output to limits/2(Vamplitude)
  Abs/1 -> V-by-f/1
  Position Generator/1 -> 3-Phase Sine Voltage Generator/2  "Eps"

== system mcb_open_loop_control_f28035_DRV8312/Open Loop Control/Codegen/Data Serial Output/Data ==
  Data : Inport
  Data_width : Inport  Port=2
  Action Port : ActionPort  ActionPortLabel=else
  Mux : Mux  Inputs=2
  Start : Constant  Value=hex2dec('0000')  OutDataTypeStr=uint16
  Data_out : Outport  VectorParamsAs1DForOutWhenUnconnected=off
  Iteration : Outport  Port=2  VectorParamsAs1DForOutWhenUnconnected=off
  wires:
  Start/1 -> Mux/2
  Mux/1 -> Data_out/1
  Data/1 -> Mux/1
  Data_width/1 -> Iteration/1

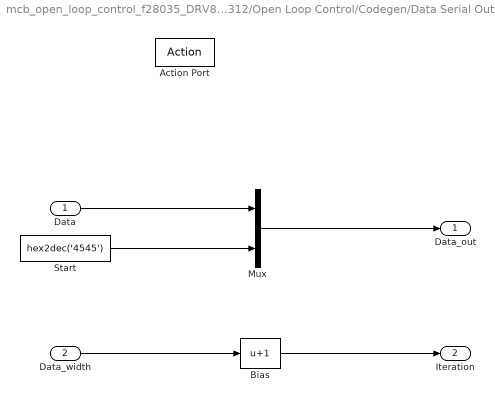
== system mcb_open_loop_control_f28035_DRV8312/Open Loop Control/Codegen/Data Serial Output/End ==
  Data : Inport
  Data_width : Inport  Port=2
  Action Port : ActionPort  ActionPortLabel=elseif(u1 == 599)
  Bias : Bias  Bias=1
  Mux : Mux  Inputs=2
  Start : Constant  Value=hex2dec('4545')  OutDataTypeStr=uint16
  Data_out : Outport  VectorParamsAs1DForOutWhenUnconnected=off
  Iteration : Outport  Port=2  VectorParamsAs1DForOutWhenUnconnected=off
  wires:
  Mux/1 -> Data_out/1
  Data_width/1 -> Bias/1
  Start/1 -> Mux/2
  Bias/1 -> Iteration/1
  Data/1 -> Mux/1

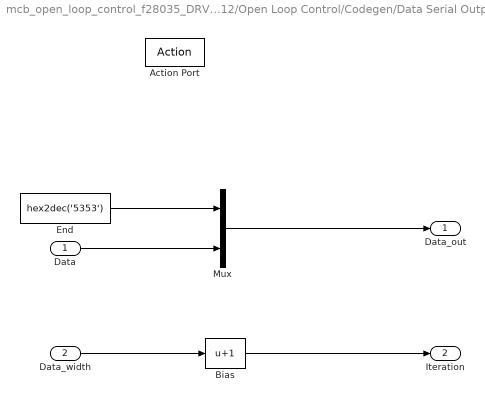
== system mcb_open_loop_control_f28035_DRV8312/Open Loop Control/Codegen/Data Serial Output/Start ==
  Data : Inport
  Data_width : Inport  Port=2
  Action Port : ActionPort  ActionPortLabel=if(u1 == 0)
  Bias : Bias  Bias=1
  End : Constant  Value=hex2dec('5353')  OutDataTypeStr=uint16
  Mux : Mux  Inputs=2
  Data_out : Outport  VectorParamsAs1DForOutWhenUnconnected=off
  Iteration : Outport  Port=2  VectorParamsAs1DForOutWhenUnconnected=off
  wires:
  End/1 -> Mux/1
  Mux/1 -> Data_out/1
  Data_width/1 -> Bias/1
  Bias/1 -> Iteration/1
  Data/1 -> Mux/2

== system mcb_open_loop_control_f28035_DRV8312/Open Loop Control/Codegen/Data Serial Output/While Iterator Subsystem ==
  Data : Inport
  Iteration : Inport  Port=2
  Add : Sum  Inputs=+-  OutDataTypeStr=Inherit: Same as first input
  Index Vector : MultiPortSwitch  Inputs=1
  SCI Transmit : c280xlib/SCI Transmit  sciModule=A  dataHead=''  dataTail=''  postInterrupt=off  numFifo=1
  While Iterator : WhileIterator  MaxIters=-1  WhileBlockType=do-while  ShowIterationPort=on  OutputDataType=int16
  wires:
  Iteration/1 -> Add/1
  Add/1 -> While Iterator/1
  Index Vector/1 -> SCI Transmit/1
  Data/1 -> Index Vector/2
  While Iterator/1 -> Index Vector/1, Add/2

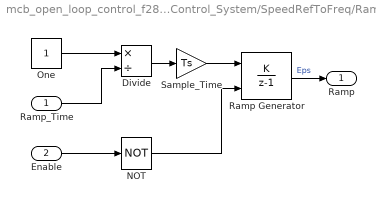
== system mcb_open_loop_control_f28035_DRV8312/Open Loop Control/Control_System/SpeedRefToFreq/Ramp Generator ==
  Ramp_Time : Inport
  Enable : Inport  Port=2
  Divide : Product  Inputs=*/  RndMeth=Simplest  OutDataTypeStr=Inherit: Same as first input
  NOT : Logic  Operator=NOT  IconShape=distinctive  AllPortsSameDT=off  OutDataTypeStr=boolean
  One : Constant  OutDataTypeStr=dataType  SampleTime=-1
  Ramp Generator : DiscreteIntegrator  IntegratorMethod=Accumulation: Forward Euler  gainval=1  ExternalReset=sampled level  SampleTime=-1  OutDataTypeStr=dataType  RndMeth=Simplest  LimitOutput=on  UpperSaturationLimit=1  LowerSaturationLimit=0  ICPrevOutput=DiscIntNeverNeededParam  ICPrevScaledInput=DiscIntNeverNeededParam
  Sample_Time : Gain  Gain=Ts  RndMeth=Simplest  OutDataTypeStr=Inherit: Same as input
  Ramp : Outport
  wires:
  Divide/1 -> Sample_Time/1
  Ramp Generator/1 -> Ramp/1  "Eps"
  Sample_Time/1 -> Ramp Generator/1
  One/1 -> Divide/1
  Ramp_Time/1 -> Divide/2
  Enable/1 -> NOT/1
  NOT/1 -> Ramp Generator/2

== system mcb_open_loop_control_f28035_DRV8312/Open Loop Control/Control_System/VabcCalc/Saturate output to limits ==
  Lower Saturation : Inport
  Vamplitude : Inport  Port=2
  Relational Operator : RelationalOperator  Operator=>  OutDataTypeStr=boolean  RndMeth=Simplest
  Saturation : Saturate  UpperLimit=0.95  LowerLimit=0  RndMeth=Simplest
  Switch : Switch  Criteria=u2 > Threshold
  Amplitude : Outport
  wires:
  Lower Saturation/1 -> Switch/3, Relational Operator/2
  Saturation/1 -> Amplitude/1
  Switch/1 -> Saturation/1
  Relational Operator/1 -> Switch/2
  Vamplitude/1 -> Switch/1, Relational Operator/1
